simulink model "c960x4096_x14_7_r2013b_frb"  (R2013b)
settings: Solver=ode45  StartTime=0.0  StopTime=40960  RelTol=1e-3
undefined symbols (not defined in the file): sfp
libraries: xbsIndex_r4 x14620, casper_library_misc x61, dspsigops x32, casper_library_multipliers x24, simulink x18, xps_library x18
(part 10 of 79)

== system c960x4096_x14_7_r2013b_frb/ds_to_tgbe/M_SYNC_TREE ==
  In1 : Inport
  Register{1..6} (6 alike) : xbsIndex_r4/Register  init=0  rst=off  en=off  dbl_ovrd=off  block_type=register
      settings: block_version=11.4
  Out1 : Outport
  Out2 : Outport  Port=2
  wires:
  Register1/1 -> Register2/1
  In1/1 -> Register1/1
  Register4/1 -> Register3/1
  Register6/1 -> Register5/1
  Register2/1 -> Register4/1, Register6/1
  Register3/1 -> Out1/1
  Register5/1 -> Out2/1

== system c960x4096_x14_7_r2013b_frb/ds_to_tgbe/NCHAN_TREE ==
  In1 : Inport
  Register{41..43,45..47} (6 alike) : xbsIndex_r4/Register  init=0  rst=off  en=off  dbl_ovrd=off  block_type=register
      settings: block_version=11.4
  Out1 : Outport
  Out2 : Outport  Port=2
  wires:
  Register41/1 -> Register42/1
  Register45/1 -> Register43/1
  Register47/1 -> Register46/1
  Register42/1 -> Register47/1, Register45/1
  Register43/1 -> Out1/1
  Register46/1 -> Out2/1
  In1/1 -> Register41/1

== system c960x4096_x14_7_r2013b_frb/ds_to_tgbe/mb1 ==
  DIN_0 : Inport
  DIN_1 : Inport  Port=2
  DIN_2 : Inport  Port=3
  DIN_3 : Inport  Port=4
  W_ADDR : Inport  Port=5
  R_ADDR : Inport  Port=6
  WE_0 : Inport  Port=7
  WE_1 : Inport  Port=8
  WE_2 : Inport  Port=9
  WE_3 : Inport  Port=10
  WE_4 : Inport  Port=11
  WE_5 : Inport  Port=12
  WE_6 : Inport  Port=13
  WE_7 : Inport  Port=14
  MUX_SEL : Inport  Port=15
  D_DIST_0 : Subsystem
  D_DIST_1 : Subsystem
  D_DIST_2 : Subsystem
  D_DIST_3 : Subsystem
  Delay{,1..7} (8 alike) : xbsIndex_r4/Delay  rst=off  infoeditControl=Selection of Reset will increase slice count due to use of real FFs and instead of SRLs  en=off  latency=1  dbl_ovrd=off  reg_retiming=off  block_type=delay
  MUX_SEL_DIST : Subsystem
  R_ADDR_DIST : Subsystem
  mb_0 : Subsystem
  mb_1 : Subsystem
  mb_2 : Subsystem
  mb_3 : Subsystem
  mb_4 : Subsystem
  mb_5 : Subsystem
  mb_6 : Subsystem
  mb_7 : Subsystem
  DOUT_0 : Outport
  DOUT_1 : Outport  Port=2
  DOUT_2 : Outport  Port=3
  DOUT_3 : Outport  Port=4
  DOUT_4 : Outport  Port=5
  DOUT_5 : Outport  Port=6
  DOUT_6 : Outport  Port=7
  DOUT_7 : Outport  Port=8
  wires:
  Delay7/1 -> DOUT_7/1
  Delay6/1 -> DOUT_6/1
  Delay5/1 -> DOUT_5/1
  Delay4/1 -> DOUT_4/1
  Delay3/1 -> DOUT_3/1
  Delay2/1 -> DOUT_2/1
  Delay1/1 -> DOUT_1/1
  Delay/1 -> DOUT_0/1
  MUX_SEL/1 -> [MUX_SEL]
  WE_7/1 -> [WE_7]
  WE_6/1 -> [WE_6]
  WE_5/1 -> [WE_5]
  WE_4/1 -> [WE_4]
  WE_3/1 -> [WE_3]
  WE_2/1 -> [WE_2]
  WE_1/1 -> [WE_1]
  WE_0/1 -> [WE_0]
  R_ADDR/1 -> [R_ADDR]
  W_ADDR/1 -> [W_ADDR]
  DIN_3/1 -> [DIN_3]
  DIN_2/1 -> [DIN_2]
  DIN_1/1 -> [DIN_1]
  DIN_0/1 -> [DIN_0]
  [R_ADDR_7] -> mb_7/6(R_ADDR)
  mb_7/1(DOUT) -> [DOUT_7]
  [MUX_SEL_7] -> mb_7/8(MUX_SEL)
  [WE_7] -> mb_7/7(WE)
  [W_ADDR] -> mb_7/5(W_ADDR)
  [DIN_3_7] -> mb_7/4(DIN_3)
  [DIN_2_7] -> mb_7/3(DIN_2)
  [DIN_1_7] -> mb_7/2(DIN_1)
  [DIN_0_7] -> mb_7/1(DIN_0)
  [R_ADDR_6] -> mb_6/6(R_ADDR)
  mb_6/1(DOUT) -> [DOUT_6]
  [MUX_SEL_6] -> mb_6/8(MUX_SEL)
  [WE_6] -> mb_6/7(WE)
  [W_ADDR] -> mb_6/5(W_ADDR)
  [DIN_3_6] -> mb_6/4(DIN_3)
  [DIN_2_6] -> mb_6/3(DIN_2)
  [DIN_1_6] -> mb_6/2(DIN_1)
  [DIN_0_6] -> mb_6/1(DIN_0)
  [R_ADDR_5] -> mb_5/6(R_ADDR)
  mb_5/1(DOUT) -> [DOUT_5]
  [MUX_SEL_5] -> mb_5/8(MUX_SEL)
  [WE_5] -> mb_5/7(WE)
  [W_ADDR] -> mb_5/5(W_ADDR)
  [DIN_3_5] -> mb_5/4(DIN_3)
  [DIN_2_5] -> mb_5/3(DIN_2)
  [DIN_1_5] -> mb_5/2(DIN_1)
  [DIN_0_5] -> mb_5/1(DIN_0)
  [R_ADDR_4] -> mb_4/6(R_ADDR)
  mb_4/1(DOUT) -> [DOUT_4]
  [MUX_SEL_4] -> mb_4/8(MUX_SEL)
  [WE_4] -> mb_4/7(WE)
  [W_ADDR] -> mb_4/5(W_ADDR)
  [DIN_3_4] -> mb_4/4(DIN_3)
  [DIN_2_4] -> mb_4/3(DIN_2)
  [DIN_1_4] -> mb_4/2(DIN_1)
  [DIN_0_4] -> mb_4/1(DIN_0)
  [R_ADDR_3] -> mb_3/6(R_ADDR)
  mb_3/1(DOUT) -> [DOUT_3]
  [MUX_SEL_3] -> mb_3/8(MUX_SEL)
  [WE_3] -> mb_3/7(WE)
  [W_ADDR] -> mb_3/5(W_ADDR)
  [DIN_3_3] -> mb_3/4(DIN_3)
  [DIN_2_3] -> mb_3/3(DIN_2)
  [DIN_1_3] -> mb_3/2(DIN_1)
  [DIN_0_3] -> mb_3/1(DIN_0)
  [R_ADDR_2] -> mb_2/6(R_ADDR)
  mb_2/1(DOUT) -> [DOUT_2]
  [MUX_SEL_2] -> mb_2/8(MUX_SEL)
  [WE_2] -> mb_2/7(WE)
  [W_ADDR] -> mb_2/5(W_ADDR)
  [DIN_3_2] -> mb_2/4(DIN_3)
  [DIN_2_2] -> mb_2/3(DIN_2)
  [DIN_1_2] -> mb_2/2(DIN_1)
  [DIN_0_2] -> mb_2/1(DIN_0)
  [R_ADDR_1] -> mb_1/6(R_ADDR)
  mb_1/1(DOUT) -> [DOUT_1]
  [MUX_SEL_1] -> mb_1/8(MUX_SEL)
  [WE_1] -> mb_1/7(WE)
  [W_ADDR] -> mb_1/5(W_ADDR)
  [DIN_3_1] -> mb_1/4(DIN_3)
  [DIN_2_1] -> mb_1/3(DIN_2)
  [DIN_1_1] -> mb_1/2(DIN_1)
  [DIN_0_1] -> mb_1/1(DIN_0)
  [R_ADDR_0] -> mb_0/6(R_ADDR)
  [DOUT_7] -> Delay7/1
  [DOUT_6] -> Delay6/1
  [DOUT_5] -> Delay5/1
  [DOUT_4] -> Delay4/1
  [DOUT_3] -> Delay3/1
  [DOUT_2] -> Delay2/1
  [DOUT_1] -> Delay1/1
  [DOUT_0] -> Delay/1
  mb_0/1(DOUT) -> [DOUT_0]
  [MUX_SEL_0] -> mb_0/8(MUX_SEL)
  [WE_0] -> mb_0/7(WE)
  [W_ADDR] -> mb_0/5(W_ADDR)
  [DIN_3_0] -> mb_0/4(DIN_3)
  [DIN_2_0] -> mb_0/3(DIN_2)
  [DIN_1_0] -> mb_0/2(DIN_1)
  [DIN_0_0] -> mb_0/1(DIN_0)
  [DIN_0] -> D_DIST_0/1(In1)
  D_DIST_0/1(Out1) -> [DIN_0_0]
  D_DIST_0/2(Out2) -> [DIN_0_1]
  D_DIST_0/3(Out3) -> [DIN_0_2]
  D_DIST_0/4(Out4) -> [DIN_0_3]
  D_DIST_0/5(Out5) -> [DIN_0_4]
  D_DIST_0/6(Out6) -> [DIN_0_5]
  D_DIST_0/7(Out7) -> [DIN_0_6]
  D_DIST_0/8(Out8) -> [DIN_0_7]
  [DIN_1] -> D_DIST_1/1(In1)
  D_DIST_1/1(Out1) -> [DIN_1_0]
  D_DIST_1/2(Out2) -> [DIN_1_1]
  D_DIST_1/3(Out3) -> [DIN_1_2]
  D_DIST_1/4(Out4) -> [DIN_1_3]
  D_DIST_1/5(Out5) -> [DIN_1_4]
  D_DIST_1/6(Out6) -> [DIN_1_5]
  D_DIST_1/7(Out7) -> [DIN_1_6]
  D_DIST_1/8(Out8) -> [DIN_1_7]
  [DIN_2] -> D_DIST_2/1(In1)
  D_DIST_2/1(Out1) -> [DIN_2_0]
  D_DIST_2/2(Out2) -> [DIN_2_1]
  D_DIST_2/3(Out3) -> [DIN_2_2]
  D_DIST_2/4(Out4) -> [DIN_2_3]
  D_DIST_2/5(Out5) -> [DIN_2_4]
  D_DIST_2/6(Out6) -> [DIN_2_5]
  D_DIST_2/7(Out7) -> [DIN_2_6]
  D_DIST_2/8(Out8) -> [DIN_2_7]
  [DIN_3] -> D_DIST_3/1(In1)
  D_DIST_3/1(Out1) -> [DIN_3_0]
  D_DIST_3/2(Out2) -> [DIN_3_1]
  D_DIST_3/3(Out3) -> [DIN_3_2]
  D_DIST_3/4(Out4) -> [DIN_3_3]
  D_DIST_3/5(Out5) -> [DIN_3_4]
  D_DIST_3/6(Out6) -> [DIN_3_5]
  D_DIST_3/7(Out7) -> [DIN_3_6]
  D_DIST_3/8(Out8) -> [DIN_3_7]
  [R_ADDR] -> R_ADDR_DIST/1(In1)
  [MUX_SEL] -> MUX_SEL_DIST/1(In1)
  MUX_SEL_DIST/1(Out1) -> [MUX_SEL_0]
  MUX_SEL_DIST/2(Out2) -> [MUX_SEL_1]
  MUX_SEL_DIST/3(Out3) -> [MUX_SEL_2]
  MUX_SEL_DIST/4(Out4) -> [MUX_SEL_3]
  MUX_SEL_DIST/5(Out5) -> [MUX_SEL_4]
  MUX_SEL_DIST/6(Out6) -> [MUX_SEL_5]
  MUX_SEL_DIST/7(Out7) -> [MUX_SEL_6]
  MUX_SEL_DIST/8(Out8) -> [MUX_SEL_7]
  R_ADDR_DIST/1(Out1) -> [R_ADDR_0]
  R_ADDR_DIST/2(Out2) -> [R_ADDR_1]
  R_ADDR_DIST/3(Out3) -> [R_ADDR_2]
  R_ADDR_DIST/4(Out4) -> [R_ADDR_3]
  R_ADDR_DIST/5(Out5) -> [R_ADDR_4]
  R_ADDR_DIST/6(Out6) -> [R_ADDR_5]
  R_ADDR_DIST/7(Out7) -> [R_ADDR_6]
  R_ADDR_DIST/8(Out8) -> [R_ADDR_7]

== system c960x4096_x14_7_r2013b_frb/ds_to_tgbe/mb_rd ==
  MSYNC : Inport
  NCHAN : Inport  Port=2
  WE_0 : Inport  Port=3
  WE_1 : Inport  Port=4
  WE_2 : Inport  Port=5
  WE_3 : Inport  Port=6
  WE_4 : Inport  Port=7
  WE_5 : Inport  Port=8
  WE_6 : Inport  Port=9
  WE_7 : Inport  Port=10
  DIN_0 : Inport  Port=11
  DIN_1 : Inport  Port=12
  DIN_2 : Inport  Port=13
  DIN_3 : Inport  Port=14
  DIN_4 : Inport  Port=15
  DIN_5 : Inport  Port=16
  DIN_6 : Inport  Port=17
  DIN_7 : Inport  Port=18
  Concat : xbsIndex_r4/Concat  num_inputs=8  dbl_ovrd=off  block_type=concat
  Concat1 : xbsIndex_r4/Concat  num_inputs=8  dbl_ovrd=off  block_type=concat
  FEC : xbsIndex_r4/Constant  const=0  gui_display_data_type=Fixed-point  arith_type=Unsigned  n_bits=64  bin_pt=0  preci_type=Single  exp_width=8  frac_width=24  explicit_period=on  period=1  equ=P=C  opselect=C  inp2=PCIN>>17  opr=+  inp1=P  carry=CIN  dbl_ovrd=off  block_type=constant
  IFG0 : xbsIndex_r4/Constant  const=12297829382473034410  gui_display_data_type=Fixed-point  arith_type=Unsigned  n_bits=64  bin_pt=0  preci_type=Single  exp_width=8  frac_width=24  explicit_period=on  period=1  equ=P=C  opselect=C  inp2=PCIN>>17  opr=+  inp1=P  carry=CIN  dbl_ovrd=off  block_type=constant
  IFG1 : xbsIndex_r4/Constant  const=12297829382473034410  gui_display_data_type=Fixed-point  arith_type=Unsigned  n_bits=64  bin_pt=0  preci_type=Single  exp_width=8  frac_width=24  explicit_period=on  period=1  equ=P=C  opselect=C  inp2=PCIN>>17  opr=+  inp1=P  carry=CIN  dbl_ovrd=off  block_type=constant
  MSYNC_TREE : Subsystem
  NCHAN_TREE : Subsystem
  NODE_0 : xbsIndex_r4/Constant  const=0  gui_display_data_type=Fixed-point  arith_type=Unsigned  n_bits=8  bin_pt=0  preci_type=Single  exp_width=8  frac_width=24  explicit_period=off  period=1  equ=P=C  opselect=C  inp2=PCIN>>17  opr=+  inp1=P  carry=CIN  dbl_ovrd=off  block_type=constant
  NODE_1 : xbsIndex_r4/Constant  const=1  gui_display_data_type=Fixed-point  arith_type=Unsigned  n_bits=8  bin_pt=0  preci_type=Single  exp_width=8  frac_width=24  explicit_period=off  period=1  equ=P=C  opselect=C  inp2=PCIN>>17  opr=+  inp1=P  carry=CIN  dbl_ovrd=off  block_type=constant
  NODE_2 : xbsIndex_r4/Constant  const=2  gui_display_data_type=Fixed-point  arith_type=Unsigned  n_bits=8  bin_pt=0  preci_type=Single  exp_width=8  frac_width=24  explicit_period=off  period=1  equ=P=C  opselect=C  inp2=PCIN>>17  opr=+  inp1=P  carry=CIN  dbl_ovrd=off  block_type=constant
  NODE_3 : xbsIndex_r4/Constant  const=3  gui_display_data_type=Fixed-point  arith_type=Unsigned  n_bits=8  bin_pt=0  preci_type=Single  exp_width=8  frac_width=24  explicit_period=off  period=1  equ=P=C  opselect=C  inp2=PCIN>>17  opr=+  inp1=P  carry=CIN  dbl_ovrd=off  block_type=constant
  NODE_4 : xbsIndex_r4/Constant  const=4  gui_display_data_type=Fixed-point  arith_type=Unsigned  n_bits=8  bin_pt=0  preci_type=Single  exp_width=8  frac_width=24  explicit_period=off  period=1  equ=P=C  opselect=C  inp2=PCIN>>17  opr=+  inp1=P  carry=CIN  dbl_ovrd=off  block_type=constant
  NODE_5 : xbsIndex_r4/Constant  const=5  gui_display_data_type=Fixed-point  arith_type=Unsigned  n_bits=8  bin_pt=0  preci_type=Single  exp_width=8  frac_width=24  explicit_period=off  period=1  equ=P=C  opselect=C  inp2=PCIN>>17  opr=+  inp1=P  carry=CIN  dbl_ovrd=off  block_type=constant
  NODE_6 : xbsIndex_r4/Constant  const=6  gui_display_data_type=Fixed-point  arith_type=Unsigned  n_bits=8  bin_pt=0  preci_type=Single  exp_width=8  frac_width=24  explicit_period=off  period=1  equ=P=C  opselect=C  inp2=PCIN>>17  opr=+  inp1=P  carry=CIN  dbl_ovrd=off  block_type=constant
  NODE_7 : xbsIndex_r4/Constant  const=7  gui_display_data_type=Fixed-point  arith_type=Unsigned  n_bits=8  bin_pt=0  preci_type=Single  exp_width=8  frac_width=24  explicit_period=off  period=1  equ=P=C  opselect=C  inp2=PCIN>>17  opr=+  inp1=P  carry=CIN  dbl_ovrd=off  block_type=constant
  XFER_0 : Subsystem
  XFER_1 : Subsystem
  XFER_2 : Subsystem
  XFER_3 : Subsystem
  XFER_4 : Subsystem
  XFER_5 : Subsystem
  XFER_6 : Subsystem
  XFER_7 : Subsystem
  R_ADDR : Outport
  MUX_SEL : Outport  Port=2
  DOUT_0 : Outport  Port=3
  STB_0 : Outport  Port=4
  EOF_0 : Outport  Port=5
  DOUT_1 : Outport  Port=6
  STB_1 : Outport  Port=7
  EOF_1 : Outport  Port=8
  DOUT_2 : Outport  Port=9
  STB_2 : Outport  Port=10
  EOF_2 : Outport  Port=11
  DOUT_3 : Outport  Port=12
  STB_3 : Outport  Port=13
  EOF_3 : Outport  Port=14
  DOUT_4 : Outport  Port=15
  STB_4 : Outport  Port=16
  EOF_4 : Outport  Port=17
  DOUT_5 : Outport  Port=18
  STB_5 : Outport  Port=19
  EOF_5 : Outport  Port=20
  DOUT_6 : Outport  Port=21
  STB_6 : Outport  Port=22
  EOF_6 : Outport  Port=23
  DOUT_7 : Outport  Port=24
  STB_7 : Outport  Port=25
  EOF_7 : Outport  Port=26
  wires:
  IFG1/1 -> [IFG1]
  IFG0/1 -> [IFG0]
  FEC/1 -> [FEC]
  [R_ADDR_7] -> Concat/8
  [R_ADDR_6] -> Concat/7
  [R_ADDR_5] -> Concat/6
  [R_ADDR_4] -> Concat/5
  [R_ADDR_3] -> Concat/4
  [R_ADDR_2] -> Concat/3
  [R_ADDR_1] -> Concat/2
  DIN_7/1 -> [DIN_7]
  DIN_6/1 -> [DIN_6]
  DIN_5/1 -> [DIN_5]
  DIN_4/1 -> [DIN_4]
  DIN_3/1 -> [DIN_3]
  DIN_2/1 -> [DIN_2]
  DIN_1/1 -> [DIN_1]
  [EOF_7] -> EOF_7/1
  [STB_7] -> STB_7/1
  [DOUT_7] -> DOUT_7/1
  [EOF_6] -> EOF_6/1
  [STB_6] -> STB_6/1
  [DOUT_6] -> DOUT_6/1
  [EOF_5] -> EOF_5/1
  [STB_5] -> STB_5/1
  DIN_0/1 -> [DIN_0]
  [DOUT_5] -> DOUT_5/1
  [EOF_4] -> EOF_4/1
  [STB_4] -> STB_4/1
  [DOUT_4] -> DOUT_4/1
  [EOF_3] -> EOF_3/1
  [STB_3] -> STB_3/1
  [DOUT_3] -> DOUT_3/1
  [EOF_2] -> EOF_2/1
  [STB_2] -> STB_2/1
  [DOUT_2] -> DOUT_2/1
  [EOF_1] -> EOF_1/1
  [STB_1] -> STB_1/1
  [DOUT_1] -> DOUT_1/1
  [EOF_0] -> EOF_0/1
  [STB_0] -> STB_0/1
  [DOUT_0] -> DOUT_0/1
  [MUX_SEL] -> MUX_SEL/1
  [R_ADDR] -> R_ADDR/1
  WE_7/1 -> [WE_7]
  WE_6/1 -> [WE_6]
  WE_5/1 -> [WE_5]
  WE_4/1 -> [WE_4]
  WE_3/1 -> [WE_3]
  WE_2/1 -> [WE_2]
  WE_1/1 -> [WE_1]
  WE_0/1 -> [WE_0]
  NCHAN/1 -> [NCHAN]
  MSYNC/1 -> [MSYNC]
  NCHAN_TREE/1(Out1) -> [NCHAN_0]
  NCHAN_TREE/2(Out2) -> [NCHAN_1]
  NCHAN_TREE/3(Out3) -> [NCHAN_2]
  NCHAN_TREE/4(Out4) -> [NCHAN_3]
  NCHAN_TREE/5(Out5) -> [NCHAN_4]
  NCHAN_TREE/6(Out6) -> [NCHAN_5]
  NCHAN_TREE/7(Out7) -> [NCHAN_6]
  NCHAN_TREE/8(Out8) -> [NCHAN_7]
  [NCHAN] -> NCHAN_TREE/1(In1)
  [MSYNC_0] -> XFER_0/1(MSYNC)
  [NCHAN_0] -> XFER_0/2(NCHAN)
  [DIN_0] -> XFER_0/3(DIN)
  [WE_0] -> XFER_0/4(WE)
  NODE_0/1 -> XFER_0/5(NODE_ID)
  [FEC] -> XFER_0/6(FEC)
  [IFG0] -> XFER_0/7(IFG0)
  [IFG1] -> XFER_0/8(IFG1)
  XFER_0/1(R_ADDR) -> [R_ADDR_0]
  XFER_0/2(MUX_SEL) -> [MUX_SEL_0]
  XFER_0/3(DOUT) -> [DOUT_0]
  XFER_0/4(STB) -> [STB_0]
  XFER_0/5(EOF) -> [EOF_0]
  [IFG1] -> XFER_1/8(IFG1)
  [IFG0] -> XFER_1/7(IFG0)
  [FEC] -> XFER_1/6(FEC)
  NODE_1/1 -> XFER_1/5(NODE_ID)
  [WE_1] -> XFER_1/4(WE)
  [DIN_1] -> XFER_1/3(DIN)
  [NCHAN_1] -> XFER_1/2(NCHAN)
  [MSYNC_1] -> XFER_1/1(MSYNC)
  XFER_1/1(R_ADDR) -> [R_ADDR_1]
  XFER_1/2(MUX_SEL) -> [MUX_SEL_1]
  XFER_1/3(DOUT) -> [DOUT_1]
  XFER_1/4(STB) -> [STB_1]
  XFER_1/5(EOF) -> [EOF_1]
  [MSYNC_2] -> XFER_2/1(MSYNC)
  [NCHAN_2] -> XFER_2/2(NCHAN)
  [DIN_2] -> XFER_2/3(DIN)
  [WE_2] -> XFER_2/4(WE)
  NODE_2/1 -> XFER_2/5(NODE_ID)
  [FEC] -> XFER_2/6(FEC)
  [IFG0] -> XFER_2/7(IFG0)
  [IFG1] -> XFER_2/8(IFG1)
  XFER_2/1(R_ADDR) -> [R_ADDR_2]
  XFER_2/2(MUX_SEL) -> [MUX_SEL_2]
  XFER_2/3(DOUT) -> [DOUT_2]
  XFER_2/4(STB) -> [STB_2]
  XFER_2/5(EOF) -> [EOF_2]
  [MSYNC_3] -> XFER_3/1(MSYNC)
  [NCHAN_3] -> XFER_3/2(NCHAN)
  [DIN_3] -> XFER_3/3(DIN)
  [WE_3] -> XFER_3/4(WE)
  NODE_3/1 -> XFER_3/5(NODE_ID)
  [FEC] -> XFER_3/6(FEC)
  [IFG0] -> XFER_3/7(IFG0)
  [IFG1] -> XFER_3/8(IFG1)
  XFER_3/1(R_ADDR) -> [R_ADDR_3]
  XFER_3/2(MUX_SEL) -> [MUX_SEL_3]
  XFER_3/3(DOUT) -> [DOUT_3]
  XFER_3/4(STB) -> [STB_3]
  XFER_3/5(EOF) -> [EOF_3]
  [MSYNC_4] -> XFER_4/1(MSYNC)
  [NCHAN_4] -> XFER_4/2(NCHAN)
  [DIN_4] -> XFER_4/3(DIN)
  [WE_4] -> XFER_4/4(WE)
  NODE_4/1 -> XFER_4/5(NODE_ID)
  [FEC] -> XFER_4/6(FEC)
  [IFG0] -> XFER_4/7(IFG0)
  [IFG1] -> XFER_4/8(IFG1)
  XFER_4/1(R_ADDR) -> [R_ADDR_4]
  XFER_4/2(MUX_SEL) -> [MUX_SEL_4]
  XFER_4/3(DOUT) -> [DOUT_4]
  XFER_4/4(STB) -> [STB_4]
  XFER_4/5(EOF) -> [EOF_4]
  [MSYNC_5] -> XFER_5/1(MSYNC)
  [NCHAN_5] -> XFER_5/2(NCHAN)
  [DIN_5] -> XFER_5/3(DIN)
  [WE_5] -> XFER_5/4(WE)
  NODE_5/1 -> XFER_5/5(NODE_ID)
  [FEC] -> XFER_5/6(FEC)
  [IFG0] -> XFER_5/7(IFG0)
  [IFG1] -> XFER_5/8(IFG1)
  XFER_5/1(R_ADDR) -> [R_ADDR_5]
  XFER_5/2(MUX_SEL) -> [MUX_SEL_5]
  XFER_5/3(DOUT) -> [DOUT_5]
  XFER_5/4(STB) -> [STB_5]
  XFER_5/5(EOF) -> [EOF_5]
  [MSYNC_6] -> XFER_6/1(MSYNC)
  [NCHAN_6] -> XFER_6/2(NCHAN)
  [DIN_6] -> XFER_6/3(DIN)
  [WE_6] -> XFER_6/4(WE)
  NODE_6/1 -> XFER_6/5(NODE_ID)
  [FEC] -> XFER_6/6(FEC)
  [IFG0] -> XFER_6/7(IFG0)
  [IFG1] -> XFER_6/8(IFG1)
  XFER_6/1(R_ADDR) -> [R_ADDR_6]
  XFER_6/2(MUX_SEL) -> [MUX_SEL_6]
  XFER_6/3(DOUT) -> [DOUT_6]
  XFER_6/4(STB) -> [STB_6]
  XFER_6/5(EOF) -> [EOF_6]
  [NCHAN_7] -> XFER_7/2(NCHAN)
  [DIN_7] -> XFER_7/3(DIN)
  [WE_7] -> XFER_7/4(WE)
  NODE_7/1 -> XFER_7/5(NODE_ID)
  [FEC] -> XFER_7/6(FEC)
  [IFG0] -> XFER_7/7(IFG0)
  [IFG1] -> XFER_7/8(IFG1)
  XFER_7/1(R_ADDR) -> [R_ADDR_7]
  XFER_7/2(MUX_SEL) -> [MUX_SEL_7]
  XFER_7/3(DOUT) -> [DOUT_7]
  XFER_7/4(STB) -> [STB_7]
  XFER_7/5(EOF) -> [EOF_7]
  [R_ADDR_0] -> Concat/1
  Concat/1 -> [R_ADDR]
  [MUX_SEL_0] -> Concat1/1
  [MUX_SEL_1] -> Concat1/2
  [MUX_SEL_2] -> Concat1/3
  [MUX_SEL_3] -> Concat1/4
  [MUX_SEL_4] -> Concat1/5
  [MUX_SEL_5] -> Concat1/6
  [MUX_SEL_6] -> Concat1/7
  [MUX_SEL_7] -> Concat1/8
  Concat1/1 -> [MUX_SEL]
  MSYNC_TREE/1(Out1) -> [MSYNC_0]
  MSYNC_TREE/2(Out2) -> [MSYNC_1]
  MSYNC_TREE/3(Out3) -> [MSYNC_2]
  MSYNC_TREE/4(Out4) -> [MSYNC_3]
  MSYNC_TREE/5(Out5) -> [MSYNC_4]
  MSYNC_TREE/6(Out6) -> [MSYNC_5]
  MSYNC_TREE/7(Out7) -> [MSYNC_6]
  MSYNC_TREE/8(Out8) -> [MSYNC_7]
  [MSYNC] -> MSYNC_TREE/1(In1)
  [MSYNC_7] -> XFER_7/1(MSYNC)

== system c960x4096_x14_7_r2013b_frb/ds_to_tgbe/mb_wr ==
  MSYNC : Inport
  SYNC_IN : Inport  Port=2
  NCHAN : Inport  Port=3
  Constant : xbsIndex_r4/Constant  const=0  gui_display_data_type=Fixed-point  arith_type=Unsigned  n_bits=3  bin_pt=0  preci_type=Single  exp_width=8  frac_width=24  explicit_period=on  period=1  equ=P=C  opselect=C  inp2=PCIN>>17  opr=+  inp1=P  carry=CIN  dbl_ovrd=off  block_type=constant
  Constant1 : xbsIndex_r4/Constant  const=1  gui_display_data_type=Fixed-point  arith_type=Unsigned  n_bits=3  bin_pt=0  preci_type=Single  exp_width=8  frac_width=24  explicit_period=on  period=1  equ=P=C  opselect=C  inp2=PCIN>>17  opr=+  inp1=P  carry=CIN  dbl_ovrd=off  block_type=constant
  Constant2 : xbsIndex_r4/Constant  const=2  gui_display_data_type=Fixed-point  arith_type=Unsigned  n_bits=3  bin_pt=0  preci_type=Single  exp_width=8  frac_width=24  explicit_period=on  period=1  equ=P=C  opselect=C  inp2=PCIN>>17  opr=+  inp1=P  carry=CIN  dbl_ovrd=off  block_type=constant
  Constant3 : xbsIndex_r4/Constant  const=3  gui_display_data_type=Fixed-point  arith_type=Unsigned  n_bits=3  bin_pt=0  preci_type=Single  exp_width=8  frac_width=24  explicit_period=on  period=1  equ=P=C  opselect=C  inp2=PCIN>>17  opr=+  inp1=P  carry=CIN  dbl_ovrd=off  block_type=constant
  Constant4 : xbsIndex_r4/Constant  const=4  gui_display_data_type=Fixed-point  arith_type=Unsigned  n_bits=3  bin_pt=0  preci_type=Single  exp_width=8  frac_width=24  explicit_period=on  period=1  equ=P=C  opselect=C  inp2=PCIN>>17  opr=+  inp1=P  carry=CIN  dbl_ovrd=off  block_type=constant
  Constant5 : xbsIndex_r4/Constant  const=5  gui_display_data_type=Fixed-point  arith_type=Unsigned  n_bits=3  bin_pt=0  preci_type=Single  exp_width=8  frac_width=24  explicit_period=on  period=1  equ=P=C  opselect=C  inp2=PCIN>>17  opr=+  inp1=P  carry=CIN  dbl_ovrd=off  block_type=constant
  Constant6 : xbsIndex_r4/Constant  const=6  gui_display_data_type=Fixed-point  arith_type=Unsigned  n_bits=3  bin_pt=0  preci_type=Single  exp_width=8  frac_width=24  explicit_period=on  period=1  equ=P=C  opselect=C  inp2=PCIN>>17  opr=+  inp1=P  carry=CIN  dbl_ovrd=off  block_type=constant
  Constant7 : xbsIndex_r4/Constant  const=7  gui_display_data_type=Fixed-point  arith_type=Unsigned  n_bits=3  bin_pt=0  preci_type=Single  exp_width=8  frac_width=24  explicit_period=on  period=1  equ=P=C  opselect=C  inp2=PCIN>>17  opr=+  inp1=P  carry=CIN  dbl_ovrd=off  block_type=constant
  Delay{1..5,27} (6 alike) : xbsIndex_r4/Delay  rst=off  infoeditControl=Selection of Reset will increase slice count due to use of real FFs and instead of SRLs  en=off  latency=1  dbl_ovrd=off  reg_retiming=off  block_type=delay
  DocBlock : simulink/Model-Wide Utilities/DocBlock  DocumentType=Text
      content=|
      | - JMR, 05/16/13
      | Added these registers while chasing timing errors.
  Logical{,1..7} (8 alike) : xbsIndex_r4/Logical  logical_function=AND  inputs=2  en=off  latency=0  precision=Full  arith_type=Unsigned  n_bits=16  bin_pt=0  align_bp=on  dbl_ovrd=off  block_type=logical
  MB_WRITE_CNTRS : Subsystem
  MB_WRITE_SLICES : Subsystem
  Register{6..7,41..43,45..47} (8 alike) : xbsIndex_r4/Register  init=0  rst=off  en=off  dbl_ovrd=off  block_type=register
      settings: block_version=11.4
  Relational{,1..7} (8 alike) : xbsIndex_r4/Relational  mode=a=b  en=off  latency=0  dbl_ovrd=off  block_type=relational
  START_LATCH : Subsystem
  WE_DECODE_BITS : Subsystem
  W_ADDR : Outport
  WE_0 : Outport  Port=2
  WE_1 : Outport  Port=3
  WE_2 : Outport  Port=4
  WE_3 : Outport  Port=5
  WE_4 : Outport  Port=6
  WE_5 : Outport  Port=7
  WE_6 : Outport  Port=8
  WE_7 : Outport  Port=9
  wires:
  Register42/1 -> Register45/1, Register7/1, Register47/1
  Register6/1 -> [NCHAN_2]
  Register7/1 -> Register6/1
  [NCHAN] -> Register41/1
  Register46/1 -> [NCHAN_1]
  Register43/1 -> [NCHAN_0]
  Register47/1 -> Register46/1
  Register45/1 -> Register43/1
  Register41/1 -> Register42/1
  [RUN] -> Delay5/1
  MB_WRITE_SLICES/1(W_ADDR) -> Delay27/1
  WE_DECODE_BITS/1(WE_DECODE) -> Delay1/1, Delay2/1, Delay3/1, Delay4/1
  Logical7/1 -> WE_7/1
  Relational7/1 -> Logical7/1
  Logical6/1 -> WE_6/1
  Relational6/1 -> Logical6/1
  Logical5/1 -> WE_5/1
  Relational5/1 -> Logical5/1
  Logical4/1 -> WE_4/1
  Relational4/1 -> Logical4/1
  Logical3/1 -> WE_3/1
  Relational3/1 -> Logical3/1
  Logical2/1 -> WE_2/1
  Relational2/1 -> Logical2/1
  Logical1/1 -> WE_1/1
  Relational1/1 -> Logical1/1
  Logical/1 -> WE_0/1
  Relational/1 -> Logical/1
  START_LATCH/1(OUT) -> [RUN]
  [SYNC_IN] -> START_LATCH/2(SET)
  [MSYNC] -> START_LATCH/1(RESET)
  [NCHAN_1] -> WE_DECODE_BITS/2(NCHAN)
  [NCHAN_2] -> MB_WRITE_SLICES/2(NCHAN)
  [NCHAN_0] -> MB_WRITE_CNTRS/3(NCHAN)
  [RUN] -> MB_WRITE_CNTRS/2(W_START)
  SYNC_IN/1 -> [SYNC_IN]
  [MSYNC] -> MB_WRITE_CNTRS/1(RESET)
  NCHAN/1 -> [NCHAN]
  MSYNC/1 -> [MSYNC]
  MB_WRITE_CNTRS/1(ADDR_CNT) -> WE_DECODE_BITS/1(ADDR_CNT), MB_WRITE_SLICES/1(ADDR_CNT)
  Constant7/1 -> Relational7/2
  Constant6/1 -> Relational6/2
  Constant5/1 -> Relational5/2
  Constant4/1 -> Relational4/2
  Constant3/1 -> Relational3/2
  Constant2/1 -> Relational2/2
  Constant1/1 -> Relational1/2
  Constant/1 -> Relational/2
  Delay27/1 -> W_ADDR/1
  Delay1/1 -> Relational1/1, Relational/1
  Delay2/1 -> Relational3/1, Relational2/1
  Delay3/1 -> Relational5/1, Relational4/1
  Delay4/1 -> Relational7/1, Relational6/1
  Delay5/1 -> Logical7/2, Logical6/2, Logical5/2, Logical4/2, Logical3/2, Logical2/2, Logical1/2, Logical/2

== system c960x4096_x14_7_r2013b_frb/leds/Pulse_Ext ==
  in : Inport
  len : Inport  Port=2
  Constant : xbsIndex_r4/Constant  const=2  gui_display_data_type=Fixed-point  arith_type=Unsigned  n_bits=32  bin_pt=0  preci_type=Single  exp_width=8  frac_width=24  explicit_period=on  period=1  equ=P=C  opselect=C  inp2=PCIN>>17  opr=+  inp1=P  carry=CIN  dbl_ovrd=off  block_type=constant
  Counter : xbsIndex_r4/Counter  cnt_type=Free Running  cnt_to=Inf  operation=Up  start_count=0  cnt_by_val=1  arith_type=Unsigned  n_bits=32  bin_pt=0  load_pin=on  rst=off  en=on  explicit_period=on  period=1  dbl_ovrd=off  use_behavioral_HDL=off  implementation=Fabric  block_type=counter
  Logical{,1..3} (4 alike) : xbsIndex_r4/Logical  logical_function=OR  inputs=2  en=off  latency=0  precision=Full  arith_type=Unsigned  n_bits=16  bin_pt=0  align_bp=on  dbl_ovrd=off  block_type=logical
  Register : xbsIndex_r4/Register  init=0  rst=on  en=off  dbl_ovrd=off  block_type=register
  Relational : xbsIndex_r4/Relational  mode=a=b  en=off  latency=0  dbl_ovrd=off  block_type=relational
  edge_detect : Subsystem  AncestorBlock=casper_library_misc/edge_detect  mask(edge_detect){edge=Rising, polarity=Active High, x_in=[0 0.08 0.08 0.16 0.16 0.24 0.24 0.32 0.32 0.4], y_in=[-1 -1  1  1  1  1  1  1  1  1], x_out=[0.6 0.68 0.68 0.76 0.76 0.84 0.84 0.92 0.92 1], y_out=[-1 -1  1  1 -1 -1 -1 -1 -1 -1]}
      mask prompts: edge "Edge Type"; polarity "Output Polarity"; x_in "Input X Positions"; y_in "Input Y Positions"; x_out "Output X Positions"; y_out "Output Y Positions"
      mask help: Output is active for one-cycle after each edge of the specified type (i.e. rising, falling or both).
      mask init: same as c960x4096_x14_7_r2013b_frb/edge_detect2
      settings: AttributesFormatString=|
      | rising edges
      | active high
      mask Help: Output is active for one-cycle after each edge of the specified type (i.e. rising, falling, or both).  Latency is zero.
      mask TypeOptions edge: Rising | Falling | Both
      mask TypeOptions polarity: Active High | Active Low
      mask Display:
      | plot(x_in_num,0.5+y_in_num*0.2);
      | plot(x_out_num,0.5+y_out_num*0.2);
  out : Outport
  wires:
  Logical3/1 -> out/1
  Logical2/1 -> Counter/1, Logical1/2
  Relational/1 -> Register/2, Logical2/2
  len/1 -> Relational/2
  Counter/1 -> Relational/1
  Constant/1 -> Counter/2
  Logical1/1 -> Counter/3
  Register/1 -> Logical3/2, Logical/1, Logical1/1
  Logical/1 -> Register/1
  edge_detect/1(out) -> Logical3/1, Logical2/1, Logical/2
  in/1 -> edge_detect/1(in)

== system c960x4096_x14_7_r2013b_frb/leds/Pulse_Ext1 ==
  in : Inport
  len : Inport  Port=2
  Constant : xbsIndex_r4/Constant  const=2  gui_display_data_type=Fixed-point  arith_type=Unsigned  n_bits=32  bin_pt=0  preci_type=Single  exp_width=8  frac_width=24  explicit_period=on  period=1  equ=P=C  opselect=C  inp2=PCIN>>17  opr=+  inp1=P  carry=CIN  dbl_ovrd=off  block_type=constant
  Counter : xbsIndex_r4/Counter  cnt_type=Free Running  cnt_to=Inf  operation=Up  start_count=0  cnt_by_val=1  arith_type=Unsigned  n_bits=32  bin_pt=0  load_pin=on  rst=off  en=on  explicit_period=on  period=1  dbl_ovrd=off  use_behavioral_HDL=off  implementation=Fabric  block_type=counter
  Logical{,1..3} (4 alike) : xbsIndex_r4/Logical  logical_function=OR  inputs=2  en=off  latency=0  precision=Full  arith_type=Unsigned  n_bits=16  bin_pt=0  align_bp=on  dbl_ovrd=off  block_type=logical
  Register : xbsIndex_r4/Register  init=0  rst=on  en=off  dbl_ovrd=off  block_type=register
  Relational : xbsIndex_r4/Relational  mode=a=b  en=off  latency=0  dbl_ovrd=off  block_type=relational
  edge_detect : Subsystem  AncestorBlock=casper_library_misc/edge_detect  mask(edge_detect){edge=Rising, polarity=Active High, x_in=[0 0.08 0.08 0.16 0.16 0.24 0.24 0.32 0.32 0.4], y_in=[-1 -1  1  1  1  1  1  1  1  1], x_out=[0.6 0.68 0.68 0.76 0.76 0.84 0.84 0.92 0.92 1], y_out=[-1 -1  1  1 -1 -1 -1 -1 -1 -1]}
      mask prompts: edge "Edge Type"; polarity "Output Polarity"; x_in "Input X Positions"; y_in "Input Y Positions"; x_out "Output X Positions"; y_out "Output Y Positions"
      mask help: Output is active for one-cycle after each edge of the specified type (i.e. rising, falling or both).
      mask init: same as c960x4096_x14_7_r2013b_frb/edge_detect2
      settings: AttributesFormatString=|
      | rising edges
      | active high
      mask Help: Output is active for one-cycle after each edge of the specified type (i.e. rising, falling, or both).  Latency is zero.
      mask TypeOptions edge: Rising | Falling | Both
      mask TypeOptions polarity: Active High | Active Low
      mask Display:
      | plot(x_in_num,0.5+y_in_num*0.2);
      | plot(x_out_num,0.5+y_out_num*0.2);
  out : Outport
  wires:
  Logical3/1 -> out/1
  Logical2/1 -> Counter/1, Logical1/2
  Relational/1 -> Register/2, Logical2/2
  len/1 -> Relational/2
  Counter/1 -> Relational/1
  Constant/1 -> Counter/2
  Logical1/1 -> Counter/3
  Register/1 -> Logical3/2, Logical/1, Logical1/1
  Logical/1 -> Register/1
  edge_detect/1(out) -> Logical3/1, Logical2/1, Logical/2
  in/1 -> edge_detect/1(in)

== system c960x4096_x14_7_r2013b_frb/one_GbE/dest_ip ==
  sim_1 : Inport
  c960x4096_x14_7_frbout_one_GbE_dest_ip_user_data_out : xbsIndex_r4/Gateway In  gui_display_data_type=Fixed-point  arith_type=Unsigned  n_bits=32  bin_pt=0  preci_type=Single  exp_width=8  frac_width=24  quantization="Round  (unbiased: +/- Inf)"  overflow=Saturate  period=1  dbl_ovrd=off  timing_constraint=None  locs_specified=off  LOCs={}  UseAsADC=off  ADCChannel='1'  inherit_from_input=off  hdl_port=on  block_type=gatewayin
  io_delay : xbsIndex_r4/Delay  rst=off  infoeditControl=Selection of Reset will increase slice count due to use of real FFs and instead of SRLs  en=off  latency=0  dbl_ovrd=off  reg_retiming=on  block_type=delay
  reint1 : xbsIndex_r4/Reinterpret  force_arith_type=on  arith_type=Unsigned  force_bin_pt=on  bin_pt=0  block_type=reinterpret
  slice_reg : xbsIndex_r4/Slice  nbits=32  boolean_output=off  mode=Lower Bit Location + Width  bit1=0  base1=MSB of Input  bit0=0  base0=LSB of Input  dbl_ovrd=off  block_type=slice
  in_reg : Outport
  wires:
  c960x4096_x14_7_frbout_one_GbE_dest_ip_user_data_out/1 -> io_delay/1
  sim_1/1 -> c960x4096_x14_7_frbout_one_GbE_dest_ip_user_data_out/1
  io_delay/1 -> slice_reg/1
  slice_reg/1 -> reint1/1
  reint1/1 -> in_reg/1

== system c960x4096_x14_7_r2013b_frb/one_GbE/dest_port ==
  sim_1 : Inport
  c960x4096_x14_7_frbout_one_GbE_dest_port_user_data_out : xbsIndex_r4/Gateway In  gui_display_data_type=Fixed-point  arith_type=Unsigned  n_bits=32  bin_pt=0  preci_type=Single  exp_width=8  frac_width=24  quantization="Round  (unbiased: +/- Inf)"  overflow=Saturate  period=1  dbl_ovrd=off  timing_constraint=None  locs_specified=off  LOCs={}  UseAsADC=off  ADCChannel='1'  inherit_from_input=off  hdl_port=on  block_type=gatewayin
  io_delay : xbsIndex_r4/Delay  rst=off  infoeditControl=Selection of Reset will increase slice count due to use of real FFs and instead of SRLs  en=off  latency=0  dbl_ovrd=off  reg_retiming=on  block_type=delay
  reint1 : xbsIndex_r4/Reinterpret  force_arith_type=on  arith_type=Unsigned  force_bin_pt=on  bin_pt=0  block_type=reinterpret
  slice_reg : xbsIndex_r4/Slice  nbits=32  boolean_output=off  mode=Lower Bit Location + Width  bit1=0  base1=MSB of Input  bit0=0  base0=LSB of Input  dbl_ovrd=off  block_type=slice
  in_reg : Outport
  wires:
  c960x4096_x14_7_frbout_one_GbE_dest_port_user_data_out/1 -> io_delay/1
  sim_1/1 -> c960x4096_x14_7_frbout_one_GbE_dest_port_user_data_out/1
  io_delay/1 -> slice_reg/1
  slice_reg/1 -> reint1/1
  reint1/1 -> in_reg/1

== system c960x4096_x14_7_r2013b_frb/one_GbE/masker ==
  rst : Inport
  din : Inport  Port=2
  vld : Inport  Port=3
  ip : Inport  Port=4
  port : Inport  Port=5
  eof : Inport  Port=6
  enable : Inport  Port=7
  Delay{,1..4} (5 alike) : xbsIndex_r4/Delay  rst=off  infoeditControl=Selection of Reset will increase slice count due to use of real FFs and instead of SRLs  en=off  latency=1  dbl_ovrd=off  reg_retiming=off  block_type=delay
  Logical1 : xbsIndex_r4/Logical  logical_function=AND  inputs=2  en=off  latency=1  precision=Full  arith_type=Unsigned  n_bits=16  bin_pt=0  align_bp=on  dbl_ovrd=off  block_type=logical
  Logical2 : xbsIndex_r4/Logical  logical_function=AND  inputs=2  en=off  latency=0  precision=Full  arith_type=Unsigned  n_bits=16  bin_pt=0  align_bp=on  dbl_ovrd=off  block_type=logical
  Register : xbsIndex_r4/Register  init=0  rst=on  en=on  dbl_ovrd=off  block_type=register
  rst_out : Outport
  dout : Outport  Port=2
  vld_out : Outport  Port=3
  ip_out : Outport  Port=4
  port_out : Outport  Port=5
  eof_out : Outport  Port=6
  wires:
  rst/1 -> Register/2, Delay2/1
  enable/1 -> Register/1
  Register/1 -> Logical1/1
  vld/1 -> Logical2/2, Logical1/2
  Logical1/1 -> vld_out/1
  eof/1 -> Delay1/1, Logical2/1
  Logical2/1 -> Register/3
  din/1 -> Delay/1
  Delay/1 -> dout/1
  Delay1/1 -> eof_out/1
  Delay2/1 -> rst_out/1
  ip/1 -> Delay3/1
  Delay3/1 -> ip_out/1
  port/1 -> Delay4/1
  Delay4/1 -> port_out/1

== system c960x4096_x14_7_r2013b_frb/one_GbE/oge_en ==
  sim_1 : Inport
  c960x4096_x14_7_frbout_one_GbE_oge_en_user_data_out : xbsIndex_r4/Gateway In  gui_display_data_type=Fixed-point  arith_type=Unsigned  n_bits=32  bin_pt=0  preci_type=Single  exp_width=8  frac_width=24  quantization="Round  (unbiased: +/- Inf)"  overflow=Saturate  period=1  dbl_ovrd=off  timing_constraint=None  locs_specified=off  LOCs={}  UseAsADC=off  ADCChannel='1'  inherit_from_input=off  hdl_port=on  block_type=gatewayin
  io_delay : xbsIndex_r4/Delay  rst=off  infoeditControl=Selection of Reset will increase slice count due to use of real FFs and instead of SRLs  en=off  latency=0  dbl_ovrd=off  reg_retiming=on  block_type=delay
  reint1 : xbsIndex_r4/Reinterpret  force_arith_type=on  arith_type=Unsigned  force_bin_pt=on  bin_pt=0  block_type=reinterpret
  slice_reg : xbsIndex_r4/Slice  nbits=32  boolean_output=off  mode=Lower Bit Location + Width  bit1=0  base1=MSB of Input  bit0=0  base0=LSB of Input  dbl_ovrd=off  block_type=slice
  in_reg : Outport
  wires:
  c960x4096_x14_7_frbout_one_GbE_oge_en_user_data_out/1 -> io_delay/1
  sim_1/1 -> c960x4096_x14_7_frbout_one_GbE_oge_en_user_data_out/1
  io_delay/1 -> slice_reg/1
  slice_reg/1 -> reint1/1
  reint1/1 -> in_reg/1

== system c960x4096_x14_7_r2013b_frb/p0_adc/Subsystem1 ==
  In1 : Inport
  In2 : Inport  Port=2
  In3 : Inport  Port=3
  In4 : Inport  Port=4
  In5 : Inport  Port=5
  In6 : Inport  Port=6
  In7 : Inport  Port=7
  In8 : Inport  Port=8
  In9 : Inport  Port=9
  In10 : Inport  Port=10
  In11 : Inport  Port=11
  In12 : Inport  Port=12
  In13 : Inport  Port=13
  In14 : Inport  Port=14
  In15 : Inport  Port=15
  In16 : Inport  Port=16
  Delay{1..10,18..20,22..24} (16 alike) : xbsIndex_r4/Delay  rst=off  infoeditControl=Selection of Reset will increase slice count due to use of real FFs and instead of SRLs  en=off  latency=1  dbl_ovrd=off  reg_retiming=on  block_type=delay
      settings: block_version=11.4
  DocBlock : simulink/Model-Wide Utilities/DocBlock  DocumentType=Text
      content=|
      | - JMR, 04/30/13
      | Converter blocks needed to convert the ASIAA ADC output from offset
      | notation (0 - 255 corresponds to -full scale to +full scale) to 2's
      | complement (-128 to +127).  Per email from Glenn Jones, 04/17/13
  bus_create : Subsystem  AncestorBlock=casper_library_flow_control/bus_create  mask(bus_create){inputNum=16}
      mask prompts: inputNum "Number of inputs:"
      mask init:
      | bus_create_init(gcb,...
      |     'inputNum', inputNum);
  converter : Subsystem
  converter1 : Subsystem
  converter10 : Subsystem
  converter11 : Subsystem
  converter12 : Subsystem
  converter13 : Subsystem
  converter14 : Subsystem
  converter15 : Subsystem
  converter2 : Subsystem
  converter3 : Subsystem
  converter4 : Subsystem
  converter5 : Subsystem
  converter6 : Subsystem
  converter7 : Subsystem
  converter8 : Subsystem
  converter9 : Subsystem
  Out1 : Outport
  wires:
  Delay6/1 -> bus_create/16(in16)
  Delay5/1 -> bus_create/15(in15)
  Delay4/1 -> bus_create/14(in14)
  Delay3/1 -> bus_create/13(in13)
  Delay2/1 -> bus_create/12(in12)
  Delay1/1 -> bus_create/11(in11)
  Delay10/1 -> bus_create/10(in10)
  Delay8/1 -> bus_create/9(in9)
  Delay24/1 -> bus_create/8(in8)
  Delay23/1 -> bus_create/7(in7)
  Delay22/1 -> bus_create/6(in6)
  Delay20/1 -> bus_create/5(in5)
  Delay19/1 -> bus_create/4(in4)
  Delay18/1 -> bus_create/3(in3)
  Delay9/1 -> bus_create/2(in2)
  Delay7/1 -> bus_create/1(in1)
  converter7/1(s8_7) -> Delay24/1
  converter6/1(s8_7) -> Delay23/1
  converter5/1(s8_7) -> Delay22/1
  converter4/1(s8_7) -> Delay20/1
  converter3/1(s8_7) -> Delay19/1
  converter2/1(s8_7) -> Delay18/1
  converter1/1(s8_7) -> Delay9/1
  converter/1(s8_7) -> Delay7/1
  converter8/1(s8_7) -> Delay8/1
  converter9/1(s8_7) -> Delay10/1
  converter10/1(s8_7) -> Delay1/1
  converter11/1(s8_7) -> Delay2/1
  converter12/1(s8_7) -> Delay3/1
  converter13/1(s8_7) -> Delay4/1
  converter14/1(s8_7) -> Delay5/1
  converter15/1(s8_7) -> Delay6/1
  In16/1 -> converter15/1(u8_0)
  In15/1 -> converter14/1(u8_0)
  In14/1 -> converter13/1(u8_0)
  In13/1 -> converter12/1(u8_0)
  In12/1 -> converter11/1(u8_0)
  In11/1 -> converter10/1(u8_0)
  In10/1 -> converter9/1(u8_0)
  In9/1 -> converter8/1(u8_0)
  In8/1 -> converter7/1(u8_0)
  In7/1 -> converter6/1(u8_0)
  In6/1 -> converter5/1(u8_0)
  In5/1 -> converter4/1(u8_0)
  In4/1 -> converter3/1(u8_0)
  In3/1 -> converter2/1(u8_0)
  In2/1 -> converter1/1(u8_0)
  In1/1 -> converter/1(u8_0)
  bus_create/1(bus_out) -> Out1/1

== system c960x4096_x14_7_r2013b_frb/p0_adc/asiaa_adc5g1 ==
  sim_a : Inport
  sim_sync : Inport  Port=2
  bias_a : Bias  Bias=128  SaturateOnIntegerOverflow=on
  c960x4096_x14_7_frbout_p0_adc_asiaa_adc5g1_sync : xbsIndex_r4/Gateway In  gui_display_data_type=Fixed-point  arith_type=Boolean  n_bits=16  bin_pt=14  preci_type=Single  exp_width=8  frac_width=24  quantization="Round  (unbiased: +/- Inf)"  overflow=Saturate  period=1  dbl_ovrd=off  timing_constraint=None  locs_specified=off  LOCs={}  UseAsADC=off  ADCChannel='1'  inherit_from_input=off  hdl_port=on  block_type=gatewayin
  c960x4096_x14_7_frbout_p0_adc_asiaa_adc5g1_user_data_i{0..7} (8 alike) : xbsIndex_r4/Gateway In  gui_display_data_type=Fixed-point  arith_type=Unsigned  n_bits=8  bin_pt=0  preci_type=Single  exp_width=8  frac_width=24  quantization=Truncate  overflow=Wrap  period=1  dbl_ovrd=off  timing_constraint=None  locs_specified=off  LOCs={}  UseAsADC=off  ADCChannel='1'  inherit_from_input=off  hdl_port=on  block_type=gatewayin
  c960x4096_x14_7_frbout_p0_adc_asiaa_adc5g1_user_data_q{0..7} (8 alike) : xbsIndex_r4/Gateway In  gui_display_data_type=Fixed-point  arith_type=Unsigned  n_bits=8  bin_pt=0  preci_type=Single  exp_width=8  frac_width=24  quantization=Truncate  overflow=Wrap  period=1  dbl_ovrd=off  timing_constraint=None  locs_specified=off  LOCs={}  UseAsADC=off  ADCChannel='1'  inherit_from_input=off  hdl_port=on  block_type=gatewayin
  delay_a0 : Delay  InitialCondition=0  InputProcessing=Inherited
  delay_a{1..15} (15 alike) : Delay  DelayLength=1  InitialCondition=0  InputProcessing=Inherited
  downsample_a0 : dspsigops/Downsample  N=16  phase=0  RateOptions=Allow multirate processing  smode=Allow multirate  fmode=Maintain input frame size  ic=0
  downsample_a1 : dspsigops/Downsample  N=16  phase=1  RateOptions=Allow multirate processing  smode=Allow multirate  fmode=Maintain input frame size  ic=0
  downsample_a10 : dspsigops/Downsample  N=16  phase=10  RateOptions=Allow multirate processing  smode=Allow multirate  fmode=Maintain input frame size  ic=0
  downsample_a11 : dspsigops/Downsample  N=16  phase=11  RateOptions=Allow multirate processing  smode=Allow multirate  fmode=Maintain input frame size  ic=0
  downsample_a12 : dspsigops/Downsample  N=16  phase=12  RateOptions=Allow multirate processing  smode=Allow multirate  fmode=Maintain input frame size  ic=0
  downsample_a13 : dspsigops/Downsample  N=16  phase=13  RateOptions=Allow multirate processing  smode=Allow multirate  fmode=Maintain input frame size  ic=0
  downsample_a14 : dspsigops/Downsample  N=16  phase=14  RateOptions=Allow multirate processing  smode=Allow multirate  fmode=Maintain input frame size  ic=0
  downsample_a15 : dspsigops/Downsample  N=16  phase=15  RateOptions=Allow multirate processing  smode=Allow multirate  fmode=Maintain input frame size  ic=0
  downsample_a2 : dspsigops/Downsample  N=16  phase=2  RateOptions=Allow multirate processing  smode=Allow multirate  fmode=Maintain input frame size  ic=0
  downsample_a3 : dspsigops/Downsample  N=16  phase=3  RateOptions=Allow multirate processing  smode=Allow multirate  fmode=Maintain input frame size  ic=0
  downsample_a4 : dspsigops/Downsample  N=16  phase=4  RateOptions=Allow multirate processing  smode=Allow multirate  fmode=Maintain input frame size  ic=0
  downsample_a5 : dspsigops/Downsample  N=16  phase=5  RateOptions=Allow multirate processing  smode=Allow multirate  fmode=Maintain input frame size  ic=0
  downsample_a6 : dspsigops/Downsample  N=16  phase=6  RateOptions=Allow multirate processing  smode=Allow multirate  fmode=Maintain input frame size  ic=0
  downsample_a7 : dspsigops/Downsample  N=16  phase=7  RateOptions=Allow multirate processing  smode=Allow multirate  fmode=Maintain input frame size  ic=0
  downsample_a8 : dspsigops/Downsample  N=16  phase=8  RateOptions=Allow multirate processing  smode=Allow multirate  fmode=Maintain input frame size  ic=0
  downsample_a9 : dspsigops/Downsample  N=16  phase=9  RateOptions=Allow multirate processing  smode=Allow multirate  fmode=Maintain input frame size  ic=0
  gain_a : Gain  Gain=128  SaturateOnIntegerOverflow=on  OutDataTypeStr=Inherit: Same as input  ParamDataTypeStr=Inherit: Same as input
  a0 : Outport
  a1 : Outport  Port=2
  a2 : Outport  Port=3
  a3 : Outport  Port=4
  a4 : Outport  Port=5
  a5 : Outport  Port=6
  a6 : Outport  Port=7
  a7 : Outport  Port=8
  a8 : Outport  Port=9
  a9 : Outport  Port=10
  a10 : Outport  Port=11
  a11 : Outport  Port=12
  a12 : Outport  Port=13
  a13 : Outport  Port=14
  a14 : Outport  Port=15
  a15 : Outport  Port=16
  sync_out : Outport  Port=17
  wires:
  sim_a/1 -> gain_a/1
  gain_a/1 -> bias_a/1
  bias_a/1 -> downsample_a0/1, downsample_a1/1, downsample_a2/1, downsample_a3/1, downsample_a4/1, downsample_a5/1, downsample_a6/1, downsample_a7/1, downsample_a8/1, downsample_a9/1, downsample_a10/1, downsample_a11/1, downsample_a12/1, downsample_a13/1, downsample_a14/1, downsample_a15/1
  downsample_a0/1 -> delay_a0/1
  delay_a0/1 -> c960x4096_x14_7_frbout_p0_adc_asiaa_adc5g1_user_data_i0/1
  c960x4096_x14_7_frbout_p0_adc_asiaa_adc5g1_user_data_i0/1 -> a0/1
  downsample_a1/1 -> delay_a1/1
  delay_a1/1 -> c960x4096_x14_7_frbout_p0_adc_asiaa_adc5g1_user_data_i1/1
  c960x4096_x14_7_frbout_p0_adc_asiaa_adc5g1_user_data_i1/1 -> a1/1
  downsample_a2/1 -> delay_a2/1
  delay_a2/1 -> c960x4096_x14_7_frbout_p0_adc_asiaa_adc5g1_user_data_i2/1
  c960x4096_x14_7_frbout_p0_adc_asiaa_adc5g1_user_data_i2/1 -> a2/1
  downsample_a3/1 -> delay_a3/1
  delay_a3/1 -> c960x4096_x14_7_frbout_p0_adc_asiaa_adc5g1_user_data_i3/1
  c960x4096_x14_7_frbout_p0_adc_asiaa_adc5g1_user_data_i3/1 -> a3/1
  downsample_a4/1 -> delay_a4/1
  delay_a4/1 -> c960x4096_x14_7_frbout_p0_adc_asiaa_adc5g1_user_data_i4/1
  c960x4096_x14_7_frbout_p0_adc_asiaa_adc5g1_user_data_i4/1 -> a4/1
  downsample_a5/1 -> delay_a5/1
  delay_a5/1 -> c960x4096_x14_7_frbout_p0_adc_asiaa_adc5g1_user_data_i5/1
  c960x4096_x14_7_frbout_p0_adc_asiaa_adc5g1_user_data_i5/1 -> a5/1
  downsample_a6/1 -> delay_a6/1
  delay_a6/1 -> c960x4096_x14_7_frbout_p0_adc_asiaa_adc5g1_user_data_i6/1
  c960x4096_x14_7_frbout_p0_adc_asiaa_adc5g1_user_data_i6/1 -> a6/1
  downsample_a7/1 -> delay_a7/1
  delay_a7/1 -> c960x4096_x14_7_frbout_p0_adc_asiaa_adc5g1_user_data_i7/1
  c960x4096_x14_7_frbout_p0_adc_asiaa_adc5g1_user_data_i7/1 -> a7/1
  downsample_a8/1 -> delay_a8/1
  delay_a8/1 -> c960x4096_x14_7_frbout_p0_adc_asiaa_adc5g1_user_data_q0/1
  c960x4096_x14_7_frbout_p0_adc_asiaa_adc5g1_user_data_q0/1 -> a8/1
  downsample_a9/1 -> delay_a9/1
  delay_a9/1 -> c960x4096_x14_7_frbout_p0_adc_asiaa_adc5g1_user_data_q1/1
  c960x4096_x14_7_frbout_p0_adc_asiaa_adc5g1_user_data_q1/1 -> a9/1
  downsample_a10/1 -> delay_a10/1
  delay_a10/1 -> c960x4096_x14_7_frbout_p0_adc_asiaa_adc5g1_user_data_q2/1
  c960x4096_x14_7_frbout_p0_adc_asiaa_adc5g1_user_data_q2/1 -> a10/1
  downsample_a11/1 -> delay_a11/1
  delay_a11/1 -> c960x4096_x14_7_frbout_p0_adc_asiaa_adc5g1_user_data_q3/1
  c960x4096_x14_7_frbout_p0_adc_asiaa_adc5g1_user_data_q3/1 -> a11/1
  downsample_a12/1 -> delay_a12/1
  delay_a12/1 -> c960x4096_x14_7_frbout_p0_adc_asiaa_adc5g1_user_data_q4/1
  c960x4096_x14_7_frbout_p0_adc_asiaa_adc5g1_user_data_q4/1 -> a12/1
  downsample_a13/1 -> delay_a13/1
  delay_a13/1 -> c960x4096_x14_7_frbout_p0_adc_asiaa_adc5g1_user_data_q5/1
  c960x4096_x14_7_frbout_p0_adc_asiaa_adc5g1_user_data_q5/1 -> a13/1
  downsample_a14/1 -> delay_a14/1
  delay_a14/1 -> c960x4096_x14_7_frbout_p0_adc_asiaa_adc5g1_user_data_q6/1
  c960x4096_x14_7_frbout_p0_adc_asiaa_adc5g1_user_data_q6/1 -> a14/1
  downsample_a15/1 -> delay_a15/1
  delay_a15/1 -> c960x4096_x14_7_frbout_p0_adc_asiaa_adc5g1_user_data_q7/1
  c960x4096_x14_7_frbout_p0_adc_asiaa_adc5g1_user_data_q7/1 -> a15/1
  sim_sync/1 -> c960x4096_x14_7_frbout_p0_adc_asiaa_adc5g1_sync/1
  c960x4096_x14_7_frbout_p0_adc_asiaa_adc5g1_sync/1 -> sync_out/1

== system c960x4096_x14_7_r2013b_frb/p0_scale/SCALE_Re_&_Im_0 ==
  P_S : Inport
  SCALE : Inport  Port=2
  Convert : xbsIndex_r4/Convert  gui_display_data_type=Fixed-point  arith_type="Signed  (2's comp)"  n_bits=8  bin_pt=5  float_type=Single  exp_bits=8  fraction_bits=24  quantization=Truncate  overflow=Wrap  en=off  latency=0  dbl_ovrd=off  pipeline=off  block_type=convert
  Convert1 : xbsIndex_r4/Convert  gui_display_data_type=Fixed-point  arith_type="Signed  (2's comp)"  n_bits=8  bin_pt=5  float_type=Single  exp_bits=8  fraction_bits=24  quantization=Truncate  overflow=Wrap  en=off  latency=0  dbl_ovrd=off  pipeline=off  block_type=convert
  Mult : xbsIndex_r4/Mult  precision=Full  arith_type="Signed  (2's comp)"  n_bits=16  bin_pt=14  quantization=Truncate  overflow=Wrap  en=off  latency=4  dbl_ovrd=off  use_behavioral_HDL=off  opt=Speed  use_embedded=on  optimum_pipeline=off  pipeline=on  use_rpm=on  placement_style=Triangular  block_type=mult
  Mult1 : xbsIndex_r4/Mult  precision=Full  arith_type="Signed  (2's comp)"  n_bits=16  bin_pt=14  quantization=Truncate  overflow=Wrap  en=off  latency=4  dbl_ovrd=off  use_behavioral_HDL=off  opt=Speed  use_embedded=on  optimum_pipeline=off  pipeline=on  use_rpm=on  placement_style=Triangular  block_type=mult
  Reinterpret : xbsIndex_r4/Reinterpret  force_arith_type=on  arith_type="Signed  (2's comp)"  force_bin_pt=on  bin_pt=17  block_type=reinterpret
  Reinterpret1 : xbsIndex_r4/Reinterpret  force_arith_type=on  arith_type="Signed  (2's comp)"  force_bin_pt=on  bin_pt=17  block_type=reinterpret
  Slice : xbsIndex_r4/Slice  nbits=18  boolean_output=off  mode=Upper Bit Location + Width  bit1=0  base1=MSB of Input  bit0=0  base0=LSB of Input  dbl_ovrd=off  block_type=slice
  Slice1 : xbsIndex_r4/Slice  nbits=18  boolean_output=off  mode=Lower Bit Location + Width  bit1=0  base1=MSB of Input  bit0=0  base0=LSB of Input  dbl_ovrd=off  block_type=slice
  Re : Outport
  Im : Outport  Port=2
  wires:
  SCALE/1 -> Mult/2, Mult1/2
  P_S/1 -> Slice1/1, Slice/1
  Convert1/1 -> Im/1
  Convert/1 -> Re/1
  Mult1/1 -> Convert1/1
  Mult/1 -> Convert/1
  Reinterpret/1 -> Mult1/1
  Reinterpret1/1 -> Mult/1
  Slice1/1 -> Reinterpret/1
  Slice/1 -> Reinterpret1/1

== system c960x4096_x14_7_r2013b_frb/p0_scale/SCALE_Re_&_Im_1 ==
  P_S : Inport
  SCALE : Inport  Port=2
  Convert : xbsIndex_r4/Convert  gui_display_data_type=Fixed-point  arith_type="Signed  (2's comp)"  n_bits=8  bin_pt=5  float_type=Single  exp_bits=8  fraction_bits=24  quantization=Truncate  overflow=Wrap  en=off  latency=0  dbl_ovrd=off  pipeline=off  block_type=convert
  Convert1 : xbsIndex_r4/Convert  gui_display_data_type=Fixed-point  arith_type="Signed  (2's comp)"  n_bits=8  bin_pt=5  float_type=Single  exp_bits=8  fraction_bits=24  quantization=Truncate  overflow=Wrap  en=off  latency=0  dbl_ovrd=off  pipeline=off  block_type=convert
  Mult : xbsIndex_r4/Mult  precision=Full  arith_type="Signed  (2's comp)"  n_bits=16  bin_pt=14  quantization=Truncate  overflow=Wrap  en=off  latency=4  dbl_ovrd=off  use_behavioral_HDL=off  opt=Speed  use_embedded=on  optimum_pipeline=off  pipeline=on  use_rpm=on  placement_style=Triangular  block_type=mult
  Mult1 : xbsIndex_r4/Mult  precision=Full  arith_type="Signed  (2's comp)"  n_bits=16  bin_pt=14  quantization=Truncate  overflow=Wrap  en=off  latency=4  dbl_ovrd=off  use_behavioral_HDL=off  opt=Speed  use_embedded=on  optimum_pipeline=off  pipeline=on  use_rpm=on  placement_style=Triangular  block_type=mult
  Reinterpret : xbsIndex_r4/Reinterpret  force_arith_type=on  arith_type="Signed  (2's comp)"  force_bin_pt=on  bin_pt=17  block_type=reinterpret
  Reinterpret1 : xbsIndex_r4/Reinterpret  force_arith_type=on  arith_type="Signed  (2's comp)"  force_bin_pt=on  bin_pt=17  block_type=reinterpret
  Slice : xbsIndex_r4/Slice  nbits=18  boolean_output=off  mode=Upper Bit Location + Width  bit1=0  base1=MSB of Input  bit0=0  base0=LSB of Input  dbl_ovrd=off  block_type=slice
  Slice1 : xbsIndex_r4/Slice  nbits=18  boolean_output=off  mode=Lower Bit Location + Width  bit1=0  base1=MSB of Input  bit0=0  base0=LSB of Input  dbl_ovrd=off  block_type=slice
  Re : Outport
  Im : Outport  Port=2
  wires:
  SCALE/1 -> Mult/2, Mult1/2
  P_S/1 -> Slice1/1, Slice/1
  Convert1/1 -> Im/1
  Convert/1 -> Re/1
  Mult1/1 -> Convert1/1
  Mult/1 -> Convert/1
  Reinterpret/1 -> Mult1/1
  Reinterpret1/1 -> Mult/1
  Slice1/1 -> Reinterpret/1
  Slice/1 -> Reinterpret1/1
